simulink library "csu_imm_immobile_update_lib"  (R2014b)
settings: Solver=ode45  SolverMode=SingleTasking  StartTime=0.0  StopTime=10.0  RelTol=1e-3
undefined symbols (not defined in the file or in its folder): imm_acc_bias_init, imm_gibbs_init, imm_gyro_bias_init, imm_position_init, imm_quat_init, imm_velocity_init, use_imu_only
settings Model: ExtModeAutoUpdateStatusClock=off  Creator=escrane  LastModifiedBy=mstewart

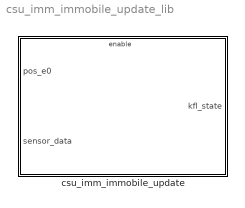
== system csu_imm_immobile_update_lib ==
  csu_imm_immobile_update : Subsystem  TreatAsAtomicUnit=on

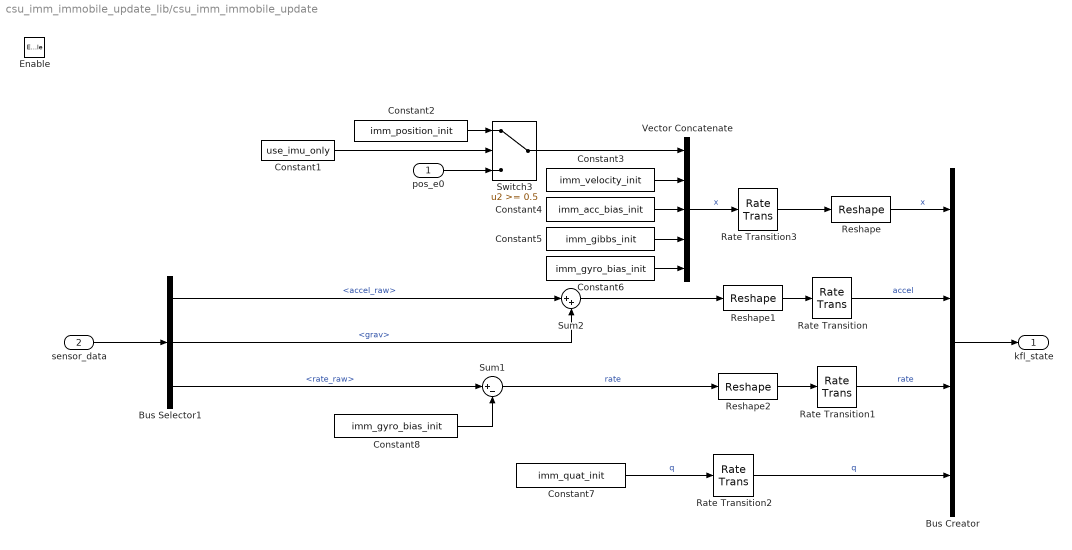
== system csu_imm_immobile_update_lib/csu_imm_immobile_update ==
  pos_e0 : Inport
  sensor_data : Inport  Port=2
  Enable : EnablePort
  Bus Creator : BusCreator
  Bus Selector1 : BusSelector  OutputSignals=accel_raw,grav,rate_raw
  Constant1 : Constant  Value=use_imu_only
  Constant2 : Constant  Value=imm_position_init
  Constant3 : Constant  Value=imm_velocity_init
  Constant4 : Constant  Value=imm_acc_bias_init
  Constant5 : Constant  Value=imm_gibbs_init
  Constant6 : Constant  Value=imm_gyro_bias_init
  Constant7 : Constant  Value=imm_quat_init
  Constant8 : Constant  Value=imm_gyro_bias_init
  Rate Transition{,1..3} (4 alike) : RateTransition  OutPortSampleTime=KF_DT
  Reshape : Reshape  OutputDimensionality=Customize  OutputDimensions=[15,1]
  Reshape1 : Reshape  OutputDimensionality=Customize  OutputDimensions=[3,1]
  Reshape2 : Reshape  OutputDimensionality=Customize  OutputDimensions=[3,1]
  Sum1 : Sum  Inputs=|+-
  Sum2 : Sum  Inputs=|++
  Switch3 : Switch  Threshold=0.5
  Vector Concatenate : Concatenate  NumInputs=5
  kfl_state : Outport
  wires:
  Bus Selector1/2 -> Sum2/2  "<grav>"
  Sum2/1 -> Reshape1/1
  Reshape2/1 -> Rate Transition1/1
  Reshape1/1 -> Rate Transition/1
  Rate Transition3/1 -> Reshape/1
  Rate Transition2/1 -> Bus Creator/4  "q"
  Rate Transition1/1 -> Bus Creator/3  "rate"
  Rate Transition/1 -> Bus Creator/2  "accel"
  Reshape/1 -> Bus Creator/1  "x"
  Constant8/1 -> Sum1/2
  Sum1/1 -> Reshape2/1  "rate"
  Bus Selector1/3 -> Sum1/1  "<rate_raw>"
  Bus Selector1/1 -> Sum2/1  "<accel_raw>"
  Constant5/1 -> Vector Concatenate/4
  Constant6/1 -> Vector Concatenate/5
  Constant4/1 -> Vector Concatenate/3
  Bus Creator/1 -> kfl_state/1
  Constant7/1 -> Rate Transition2/1  "q"
  Vector Concatenate/1 -> Rate Transition3/1  "x"
  Constant2/1 -> Switch3/1
  Constant1/1 -> Switch3/2
  pos_e0/1 -> Switch3/3
  Switch3/1 -> Vector Concatenate/1
  sensor_data/1 -> Bus Selector1/1
  Constant3/1 -> Vector Concatenate/2
